simulink model "squareroot_sim"  (R2019b)
settings: Solver=VariableStepAuto  StartTime=0.0  StopTime=1  RelTol=1e-3
settings Model: Creator=kanth  LastModifiedBy=kanth

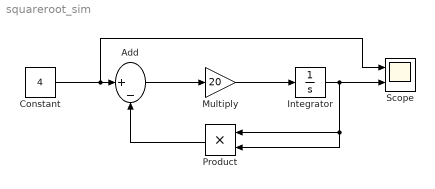
== system squareroot_sim ==
  Add : Sum  Inputs=|+-
  Constant : Constant  Value=4
  Integrator : Integrator
  Multiply : Gain  Gain=20
  Product : Product
  Scope : Scope  NumInputPorts=2
  wires:
  Constant/1 -> Scope/1, Add/1
  Add/1 -> Multiply/1
  Multiply/1 -> Integrator/1
  Product/1 -> Add/2
  Integrator/1 -> Scope/2, Product/2, Product/1
